simulink model "Expt7_DeadTime"  (R2020b)
settings: Solver=VariableStepAuto  StartTime=0.0  StopTime=200  RelTol=1e-3
settings Model: Creator=geniu  LastModifiedBy=geniu

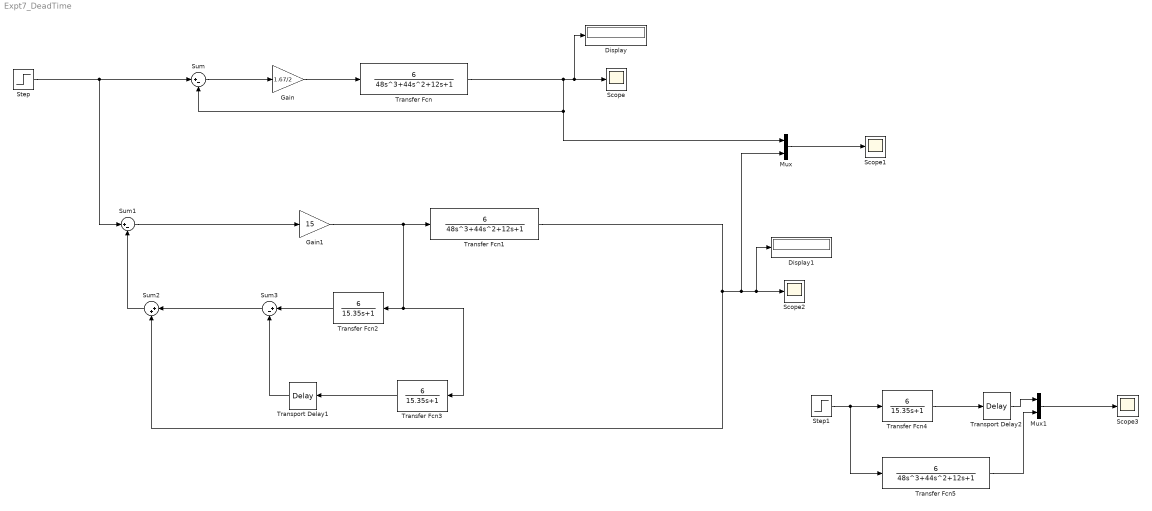
== system Expt7_DeadTime ==
  Display : Display
  Display1 : Display
  Gain : Gain  Gain=1.67/2
  Gain1 : Gain  Gain=15
  Mux : Mux  Inputs=2
  Mux1 : Mux  Inputs=2
  Scope{,1..3} (4 alike) : Scope
  Step : Step  SampleTime=0
  Step1 : Step  SampleTime=0
  Sum : Sum  Inputs=|+-
  Sum1 : Sum  Inputs=|+-
  Sum2 : Sum  Inputs=|++
  Sum3 : Sum  Inputs=|+-
  Transfer Fcn : TransferFcn  Numerator=[6]  Denominator=[48 44 12 1]
  Transfer Fcn1 : TransferFcn  Numerator=[6]  Denominator=[48 44 12 1]
  Transfer Fcn2 : TransferFcn  Numerator=[6]  Denominator=[15.35 1]
  Transfer Fcn3 : TransferFcn  Numerator=[6]  Denominator=[15.35 1]
  Transfer Fcn4 : TransferFcn  Numerator=[6]  Denominator=[15.35 1]
  Transfer Fcn5 : TransferFcn  Numerator=[6]  Denominator=[48 44 12 1]
  Transport Delay1 : TransportDelay  DelayTime=2.71
  Transport Delay2 : TransportDelay  DelayTime=2.71
  wires:
  Gain/1 -> Transfer Fcn/1
  Transfer Fcn/1 -> Display/1, Scope/1, Mux/1, Sum/2
  Sum/1 -> Gain/1
  Step/1 -> Sum1/1, Sum/1
  Sum1/1 -> Gain1/1
  Gain1/1 -> Transfer Fcn3/1, Transfer Fcn2/1, Transfer Fcn1/1
  Mux/1 -> Scope1/1
  Transfer Fcn1/1 -> Sum2/2, Mux/2, Display1/1, Scope2/1
  Transfer Fcn2/1 -> Sum3/1
  Sum3/1 -> Sum2/1
  Transfer Fcn3/1 -> Transport Delay1/1
  Transport Delay1/1 -> Sum3/2
  Sum2/1 -> Sum1/2
  Step1/1 -> Transfer Fcn5/1, Transfer Fcn4/1
  Transfer Fcn4/1 -> Transport Delay2/1
  Mux1/1 -> Scope3/1
  Transport Delay2/1 -> Mux1/1
  Transfer Fcn5/1 -> Mux1/2
